simulink model "Stufa_stanza"  (R2022b)
settings: Solver=VariableStepAuto  StartTime=0.0  StopTime=100  RelTol=1e-3
values from neighbouring files (symbols this model uses):
  C1 = 1    [Stufa.m]
  C2 = 1    [Stufa.m]
  Q1 = 0    [Stufa.m]
  Q2 = 5    [Stufa.m]
  R1 = 1    [Stufa.m]
  R2 = 1    [Stufa.m]
  Te1 = 1    [Stufa.m]
  Te2 = 5    [Stufa.m]
settings Model: Creator=giuli  LastModifiedBy=giuli

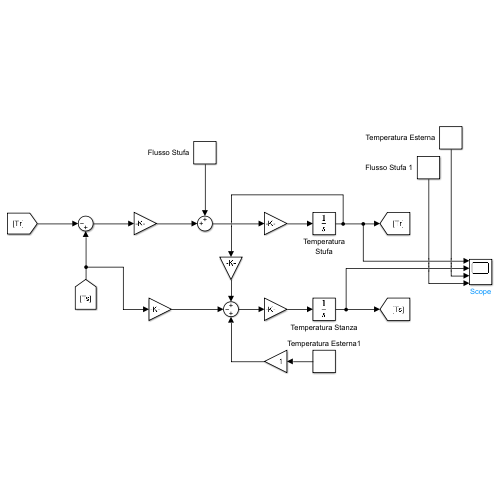
[thumbnail: Simulink's stored preview of the top-level diagram]
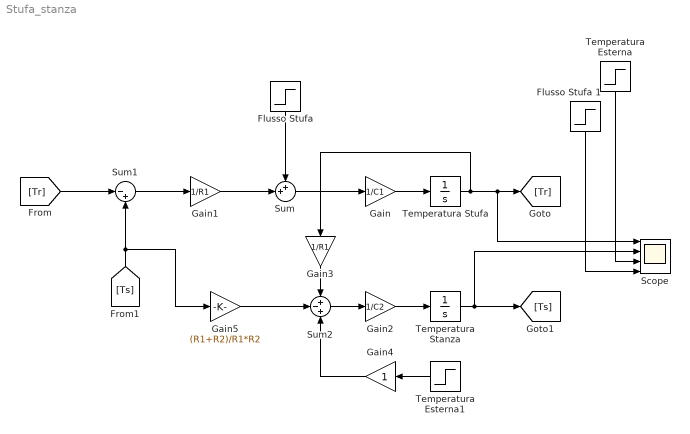
== system Stufa_stanza ==
  Flusso Stufa : Step  Time=50  Before=Q1  After=Q2  SampleTime=0.1
  Flusso Stufa 1 : Step  Time=50  Before=Q1  After=Q2  SampleTime=0
  Gain : Gain  Gain=1/C1
  Gain1 : Gain  Gain=1/R1
  Gain2 : Gain  Gain=1/C2
  Gain3 : Gain  Gain=1/R1
  Gain4 : Gain
  Gain5 : Gain  Gain=(R1+R2)/R1*R2
  Scope : Scope  NumInputPorts=4
  Sum : Sum  Inputs=++|
  Sum1 : Sum  Inputs=|-+
  Sum2 : Sum  Inputs=+-+
  Temperatura Stufa : Integrator
  Temperatura Esterna : Step  Time=25  Before=Te1  After=Te2  SampleTime=0
  Temperatura Esterna1 : Step  Time=25  Before=Te1  After=Te2  SampleTime=0
  Temperatura Stanza : Integrator
  wires:
  Gain/1 -> Temperatura Stufa/1
  Sum/1 -> Gain/1
  Gain1/1 -> Sum/2
  Sum1/1 -> Gain1/1
  Temperatura Stufa/1 -> Scope/1, [Tr], Gain3/1
  Temperatura Stanza/1 -> Scope/2, [Ts]
  Gain2/1 -> Temperatura Stanza/1
  Gain3/1 -> Sum2/1
  Sum2/1 -> Gain2/1
  Temperatura Esterna1/1 -> Gain4/1
  Gain4/1 -> Sum2/3
  [Tr] -> Sum1/1
  [Ts] -> Gain5/1, Sum1/2
  Gain5/1 -> Sum2/2
  Flusso Stufa/1 -> Sum/1
  Temperatura Esterna/1 -> Scope/3
  Flusso Stufa 1/1 -> Scope/4
